simulink model "Copy_3_continuos_plant"  (R2016b)
settings: Solver=ode15s  StartTime=0.0  StopTime=300  RelTol=0.01  AbsTol=0.01
undefined symbols (not defined in the file or in its folder): deg, rad, s
libraries: simulink x12, aerolibconvert2 x4, aerolib6dof2 x2, dspsrcs4 x2, dspinverses x1
(part 2 of 2)

== matlab function Copy_3_continuos_plant/Translational Motion Observer/error dynamics ==
  data: p_n_delta_true input; p_n_delta_err output size=[3,1]; p_n_delta_stim input; beta_true input; beta_stim input; beta_err output; v_n_true input; v_n_stim input; f_n_true input; f_n_stim input; v_n_err output; f_n_err output
function [p_n_delta_err, beta_err, v_n_err, f_n_err] = errDyn(p_n_delta_true, p_n_delta_stim, beta_true, beta_stim, v_n_true, v_n_stim, f_n_true, f_n_stim)


p_n_delta_err = p_n_delta_true - p_n_delta_stim;

beta_err = beta_true - beta_stim;

v_n_err = v_n_true - v_n_stim;

f_n_err = f_n_true - f_n_stim;

end

== matlab function Copy_3_continuos_plant/Nonlinear algebraic transform and solution/algebraic transform solution ==
  data: C_dx input; x_at output; delta input
function x_at = solAT(C_dx, delta)

% this solution is described in the Appendix
% that is correct only for m >= 5

pC_dx = pinv(C_dx);

x_at = pC_dx * (delta / 2);

end

== matlab function Copy_3_continuos_plant/algebraic transform - error dynamics/MATLAB Function ==
  data: p_n_true input; p_n_err output; beta input; x_at input; beta_err output
function [p_n_err, beta_err] = fcn(p_n_true, beta, x_at)

% from algebraic transform
p_n_stim = x_at(1:3,1);
beta_stim = x_at(4,1);

% error dynamics
p_n_err = p_n_true - p_n_stim;
beta_err = beta - beta_stim;

end
